simulink model "debug_FTMeas_shoes_legacy"  (Simulink 8.3)
settings: Solver=FixedStepDiscrete  StartTime=0.0  StopTime=inf  FixedStep=0.01  RelTol=1e-3
InitFcn:
  | ROBOT_DOF=23;
libraries: WBToolboxLibrary x9
settings Model: Creator=DanielePucci  LastModifiedBy=icub  CovSFcnEnable=on
settings DataIOCC: SaveFormat=StructureWithTime  SignalLoggingSaveFormat=Dataset
settings DebuggingCC: UnderspecifiedInitializationDetection=Simplified  MergeDetectMultiDrivingBlocksExec=error  SolverPrmCheckMsg=none  FrameProcessingCompatibilityMsg=error  StateNameClashWarn=none
settings HardwareCC: ProdBitPerPointer=64  ProdLargestAtomicFloat=Float  ProdIntDivRoundTo=Zero  ProdEndianess=LittleEndian  ProdHWDeviceType=Specified
settings GRTTargetCC: GeneratePreprocessorConditionals=Use local settings  CombineOutputUpdateFcns=on  GRTInterface=off

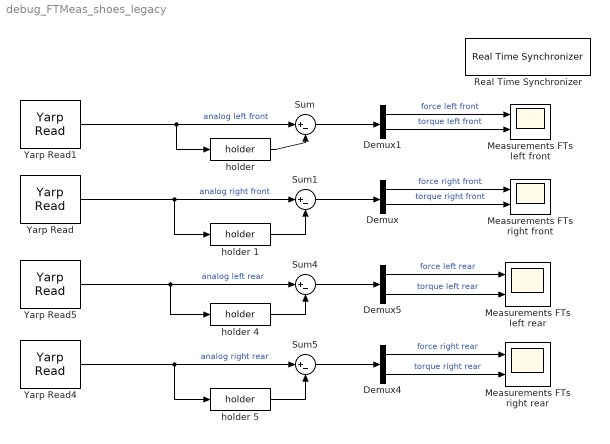
== system debug_FTMeas_shoes_legacy ==
  Demux{,1,4..5} (4 alike) : Demux  Outputs=2
  Measurements FTs left front : Scope  NumInputPorts=2
      settings: TimeRange=60  ShowLegends=on  MaxDataPoints=5000  SaveToWorkspace=off  SaveName=ScopeData2  YMin=-19.48535~-2.11395  YMax=29.67908~1.5329  SampleTime=-1
  Measurements FTs left rear : Scope  NumInputPorts=2
      settings: TimeRange=60  ShowLegends=on  MaxDataPoints=5000  SaveToWorkspace=off  YMin=-19.48535~-2.11395  YMax=29.67908~1.5329  SampleTime=-1
  Measurements FTs right front : Scope  NumInputPorts=2
      settings: TimeRange=60  ShowLegends=on  MaxDataPoints=5000  SaveToWorkspace=off  SaveName=ScopeData  YMin=-19.48535~-2.11395  YMax=29.67908~1.5329  SampleTime=-1
  Measurements FTs right rear : Scope  NumInputPorts=2
      settings: TimeRange=60  ShowLegends=on  MaxDataPoints=5000  SaveToWorkspace=off  SaveName=ScopeData4  YMin=-19.48535~-2.11395  YMax=29.67908~1.5329  SampleTime=-1
  Real Time Synchronizer : WBToolboxLibrary/Utilities/Real Time Synchronizer  period=0.01
  Sum{,1,4..5} (4 alike) : Sum  Inputs=|+-
  Yarp Read : WBToolboxLibrary/Utilities/Yarp Read  portName='ft/ftShoe_Right_Front/analog:o'  signalSize=6  timeout=0.5  blocking=off  timestamp=off  autoconnect=on  errorOnConnection=off
  Yarp Read1 : WBToolboxLibrary/Utilities/Yarp Read  portName='ft/ftShoe_Left_Front/analog:o'  signalSize=6  timeout=0.5  blocking=off  timestamp=off  autoconnect=on  errorOnConnection=off
  Yarp Read4 : WBToolboxLibrary/Utilities/Yarp Read  portName='ft/ftShoe_Right_Rear/analog:o'  signalSize=6  timeout=0.5  blocking=off  timestamp=off  autoconnect=on  errorOnConnection=off
  Yarp Read5 : WBToolboxLibrary/Utilities/Yarp Read  portName='ft/ftShoe_Left_Rear/analog:o'  signalSize=6  timeout=0.5  blocking=off  timestamp=off  autoconnect=on  errorOnConnection=off
  holder {,1,4..5} (4 alike) : WBToolboxLibrary/Utilities/holder 
  wires:
  Yarp Read/1 -> holder 1/1, Sum1/1  "analog right front"
  Demux/1 -> Measurements FTs right front/1  "force right front"
  Demux/2 -> Measurements FTs right front/2  "torque right front"
  Yarp Read1/1 -> Sum/1, "holder "/1  "analog left front"
  Demux1/1 -> Measurements FTs left front/1  "force left front"
  Demux1/2 -> Measurements FTs left front/2  "torque left front"
  "holder "/1 -> Sum/2
  Sum/1 -> Demux1/1
  holder 1/1 -> Sum1/2
  Sum1/1 -> Demux/1
  Yarp Read4/1 -> holder 5/1, Sum5/1  "analog right rear"
  Demux4/1 -> Measurements FTs right rear/1  "force right rear"
  Demux4/2 -> Measurements FTs right rear/2  "torque right rear"
  Yarp Read5/1 -> Sum4/1, holder 4/1  "analog left rear"
  Demux5/2 -> Measurements FTs left rear/2  "torque left rear"
  holder 4/1 -> Sum4/2
  Sum4/1 -> Demux5/1
  holder 5/1 -> Sum5/2
  Sum5/1 -> Demux4/1
  Demux5/1 -> Measurements FTs left rear/1  "force left rear"
